simulink model "model"  (R2020b)
settings: Solver=VariableStepAuto  StartTime=0.0  StopTime=0.04  RelTol=1e-3
values from neighbouring files (symbols this model uses):
  L = table2array(readtable('data.xlsx', 'Range','B1:B2', 'ReadRowNames',false))    [script.m]
  P_load = input('Введите мощность нагрузки в кВт: ')    [script.m]
  R0 = table2array(readtable('data.xlsx', 'Range','G1:G11', 'ReadRowNames',false))    [script.m]
  Unom = 230    [script.m]
undefined symbols (not defined in the file or in its folder): n
libraries: powerlib x7, powerlib_meascontrol x3
settings Model: Creator=1655070  LastModifiedBy=1655070

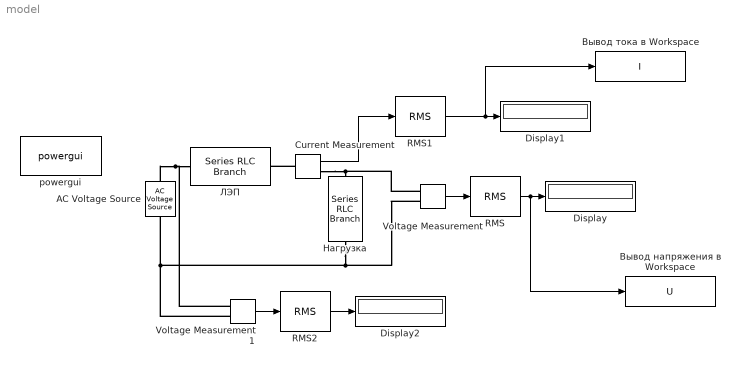
== system model ==
  AC Voltage Source : powerlib/Electrical Sources/AC Voltage Source  Amplitude=Unom*sqrt(2)  Phase=0  Frequency=50  SampleTime=0  Measurements=None  BusType=swing  Pref=10e3  Qref=0  Qmin=-inf  Qmax=+inf
  Current Measurement : powerlib/Measurements/Current Measurement  PhasorSimulation=off  OutputType=Complex  PSBequivalent=0
  Display : Display
  Display1 : Display
  Display2 : Display
  RMS : powerlib_meascontrol/Measurements/RMS  TrueRMS=on  Freq=50  RMSInit=120  Ts=0
  RMS1 : powerlib_meascontrol/Measurements/RMS  TrueRMS=on  Freq=50  RMSInit=120  Ts=0
  RMS2 : powerlib_meascontrol/Measurements/RMS  TrueRMS=on  Freq=50  RMSInit=120  Ts=0
  Voltage Measurement : powerlib/Measurements/Voltage Measurement  PhasorSimulation=off  OutputType=Complex  PSBequivalent=0
  Voltage Measurement1 : powerlib/Measurements/Voltage Measurement  PhasorSimulation=off  OutputType=Complex  PSBequivalent=0
  powergui : powerlib/powergui  Priority=1  SimulationMode=Discrete  SampleTime=50e-6  frequency=60  Iterations=50  frequencyindice=50  Pbase=100e6  ErrMax=1e-4  UnitsV=kV  UnitsW=MW  buscounter=0  FunctionMessages=off  echomessages=off  EnableUseOfTLC=off  CurrentSourceSwitches=off  DisableSnubberDevices=off  DisableRonSwitches=off  DisableVfSwitches=off  DisplayEquations=off  AutomaticDiscreteSolvers=off  SolverType=Tustin/Backward Euler (TBE)  Interpol=off  ExternalGateDelay=off  methode=off  Ts=100  x0status=blocks  SPID=on  SwTol=0  HookPort=off  NonlinearTolerance=1e-4  nMaxIteration=100  ContinueOnMaxIteration=off  RestoreLinks=warning  ResistiveCurrentMeasurement=off  Frange=[0:2:500]  Ylog=off  Xlog=on  ShowGrid=off  save=off  variable=ZData  structure=0  ZoomFFT=off  StartTime=0.0  cycles=1  DisplayStyle=1  fundamental=60  FreqAxis=off  MaxFrequency=1000  frequencyindicesteady=1  RmsSteady=1  display=off
  Вывод напряжения в Workspace : ToWorkspace  VariableName=U  SampleTime=0.04-50*1e-6
      settings: Save2DSignal=2-D array (concatenate along first dimension)
  Вывод тока в Workspace : ToWorkspace  VariableName=I  SampleTime=0.04-50*1e-6
      settings: Save2DSignal=2-D array (concatenate along first dimension)
  ЛЭП : powerlib/Elements/Series RLC Branch  LConnTagsString=__new0  RConnTagsString=__new0  BranchType=R  Resistance=2*R0(n)*L/1000  Inductance=1e-3  SetiL0=off  InitialCurrent=0  Capacitance=1e-6  Setx0=off  InitialVoltage=0  Measurements=None
  Нагрузка : powerlib/Elements/Series RLC Branch  LConnTagsString=__new0  RConnTagsString=__new0  BranchType=R  Resistance=Unom^2/P_load*1e-3  Inductance=1e-3  SetiL0=off  InitialCurrent=0  Capacitance=1e-6  Setx0=off  InitialVoltage=0  Measurements=None
  wires:
  Voltage Measurement/1 -> RMS/1
  RMS1/1 -> Вывод тока в Workspace/1, Display1/1
  Current Measurement/1 -> RMS1/1
  RMS2/1 -> Display2/1
  Voltage Measurement1/1 -> RMS2/1
  RMS/1 -> Вывод напряжения в Workspace/1, Display/1
  connections:
  AC Voltage Source/RConn1 -- Voltage Measurement1/LConn1 -- ЛЭП/LConn1
  Нагрузка/RConn1 -- Voltage Measurement/LConn2 -- AC Voltage Source/LConn1 -- Voltage Measurement1/LConn2
  Current Measurement/LConn1 -- ЛЭП/RConn1
  Current Measurement/RConn1 -- Нагрузка/LConn1 -- Voltage Measurement/LConn1
